simulink model "LCK_0112"  (R2018b)
settings: Solver=FixedStepDiscrete  StartTime=0.0  StopTime=inf  FixedStep=0.01  RelTol=1e-3
PostLoadFcn:
  | if any(exist('dsrtsu_mdlpostloadfcn', 'file') ~= 0), dsrtsu_mdlpostloadfcn('Execute', bdroot); end
values from neighbouring files (symbols this model uses):
  C_DEG2RAD = 0.0175    [LCK_Macro.sldd]
  C_KPH2MPS = 0.2778    [LCK_Macro.sldd]
  C_NEARZERO = 0.0001    [LCK_Macro.sldd]
  C_ONE = 1.0    [LCK_Macro.sldd]
  C_RAD2DEG = 57.2958    [LCK_Macro.sldd]
  C_ZERO = 0.0    [LCK_Macro.sldd]
  k_accel_pedal_pos_per_speed_x : value not decoded    [LCK_LogicPara.sldd]
  k_accel_pedal_pos_per_speed_z : value not decoded    [LCK_LogicPara.sldd]
  k_brake_suprress_hold = 1000.0    [LCK_LogicPara.sldd]
  k_driver_appl_torque_filt = 50.0    [LCK_LogicPara.sldd]
  k_driver_suppression_hold_time = 3000.0    [LCK_LogicPara.sldd]
  k_hands_on_wheel_hold_msec = 500.0    [LCK_LogicPara.sldd]
  k_hands_on_wheel_torque_hi = 0.2    [LCK_LogicPara.sldd]
  k_hands_on_wheel_torque_lo = 0.15    [LCK_LogicPara.sldd]
  k_handsoff_delay_cycles = 50.0    [LCK_LogicPara.sldd]
  k_handsoff_torq_Lo_CR = 0.3    [LCK_LogicPara.sldd]
  k_handson_delay_cycles = 5.0    [LCK_LogicPara.sldd]
  k_HighAccel_suppress_hold = 3000.0    [LCK_LogicPara.sldd]
  k_HLR_suprress_hold = 3000.0    [LCK_LogicPara.sldd]
  k_hs_StrAng_CR_threshold_z : value not decoded    [LCK_LogicPara.sldd]
  k_LC_Exit_Switch = 0.0    [LCK_LogicPara.sldd]
  k_LCG_Configured = 1.0    [LCK_LogicPara.sldd]
  k_LCK_A0_Rdy2Act_UseConst = 0.0    [LCK_LogicPara.sldd]
  k_LCK_A0Fac_ActSta : value not decoded    [LCK_CtrlPara.sldd]
  k_LCK_A0Fac_DrvStm : value not decoded    [LCK_CtrlPara.sldd]
  k_LCK_A0Shift_LftCurv : value not decoded    [LCK_CtrlPara.sldd]
  k_LCK_A0Shift_RgtCurv : value not decoded    [LCK_CtrlPara.sldd]
  k_LCK_A0Shift_StraLan = 0.0    [LCK_CtrlPara.sldd]
  k_LCK_A0ShiftFac_Dy_LftCurv : value not decoded    [LCK_CtrlPara.sldd]
  k_LCK_A0ShiftFac_Dy_RgtCurv : value not decoded    [LCK_CtrlPara.sldd]
  k_LCK_A0ShiftFac_Vspd : value not decoded    [LCK_CtrlPara.sldd]
  k_LCK_accel_inhibit_thold = 35.0    [LCK_LogicPara.sldd]
  k_LCK_Active2Ready_Mask = 255.0    [LCK_LogicPara.sldd]
  k_LCK_CvatRateBks : value not decoded    [LCK_CtrlPara.sldd]
  k_LCK_CvatrBks : value not decoded    [LCK_CtrlPara.sldd]
  k_LCK_DFac_Dy : value not decoded    [LCK_CtrlPara.sldd]
  k_LCK_DFac_Dy_Curv : value not decoded    [LCK_CtrlPara.sldd]
  k_LCK_DFac_HaCurCen : value not decoded    [LCK_CtrlPara.sldd]
  k_LCK_DFac_HaCurSid : value not decoded    [LCK_CtrlPara.sldd]
  k_LCK_DFac_HadCurCen : value not decoded    [LCK_CtrlPara.sldd]
  k_LCK_DFac_HadCurSid : value not decoded    [LCK_CtrlPara.sldd]
  k_LCK_DFac_HadStrCen : value not decoded    [LCK_CtrlPara.sldd]
  k_LCK_DFac_HadStrSid : value not decoded    [LCK_CtrlPara.sldd]
  k_LCK_DFac_HaStrCen : value not decoded    [LCK_CtrlPara.sldd]
  k_LCK_DFac_HaStrSid : value not decoded    [LCK_CtrlPara.sldd]
  k_LCK_DFac_Rad : value not decoded    [LCK_CtrlPara.sldd]
  k_LCK_DFac_SA_CurCen : value not decoded    [LCK_CtrlPara.sldd]
  k_LCK_DFac_SA_CurSid : value not decoded    [LCK_CtrlPara.sldd]
  k_LCK_DFac_SA_StrCen : value not decoded    [LCK_CtrlPara.sldd]
  k_LCK_DFac_SA_StrSid : value not decoded    [LCK_CtrlPara.sldd]
  k_LCK_DFac_SS_CurCen : value not decoded    [LCK_CtrlPara.sldd]
  k_LCK_DFac_SS_CurSid : value not decoded    [LCK_CtrlPara.sldd]
  k_LCK_DFac_SS_StrCen : value not decoded    [LCK_CtrlPara.sldd]
  k_LCK_DFac_SS_StrSid : value not decoded    [LCK_CtrlPara.sldd]
  k_LCK_DFac_Vspd : value not decoded    [LCK_CtrlPara.sldd]
  k_LCK_DlyTm_DrvStim = 0.2    [LCK_CtrlPara.sldd]
  k_LCK_DTermMax = 2.0    [LCK_CtrlPara.sldd]
  k_LCK_DyBks_Curv : value not decoded    [LCK_CtrlPara.sldd]
  k_LCK_Enable_POOnly = 1.0    [LCK_LogicPara.sldd]
  k_LCK_Entry_DistBuffer = 0.1    [LCK_LogicPara.sldd]
  k_LCK_Fac_Vspd2RngThr_FalRec = 0.23    [LCK_CtrlPara.sldd]
  k_LCK_Ffw_CvatSwh = 0.0    [LCK_CtrlPara.sldd]
  k_LCK_Ffw_DyBks : value not decoded    [LCK_CtrlPara.sldd]
  k_LCK_Ffw_TimCon_CmdFlt = 0.0    [LCK_CtrlPara.sldd]
  k_LCK_FfwDeltaFac_Rad_Lft : value not decoded    [LCK_CtrlPara.sldd]
  k_LCK_FfwDeltaFac_Rad_Rgt : value not decoded    [LCK_CtrlPara.sldd]
  k_LCK_FfwDeltaFac_Vspd : value not decoded    [LCK_CtrlPara.sldd]
  k_LCK_FfwFac_CvatRate_Lft : value not decoded    [LCK_CtrlPara.sldd]
  k_LCK_FfwFac_CvatRate_Rgt : value not decoded    [LCK_CtrlPara.sldd]
  k_LCK_FfwFac_Dy : value not decoded    [LCK_CtrlPara.sldd]
  k_LCK_FfwFac_Rad_Lft : value not decoded    [LCK_CtrlPara.sldd]
  k_LCK_FfwFac_Rad_Rgt : value not decoded    [LCK_CtrlPara.sldd]
  k_LCK_FfwFac_Vspd : value not decoded    [LCK_CtrlPara.sldd]
  k_LCK_FfwTorq_Cvat : value not decoded    [LCK_CtrlPara.sldd]
  k_LCK_HAFac_ActSta : value not decoded    [LCK_CtrlPara.sldd]
  k_LCK_HAFac_DrvStm : value not decoded    [LCK_CtrlPara.sldd]
  k_LCK_HaloTime = 2000.0    [LCK_LogicPara.sldd]
  k_LCK_HaloTime_Switch = 0.0    [LCK_LogicPara.sldd]
  k_LCK_HARFac_ActSta : value not decoded    [LCK_CtrlPara.sldd]
  k_LCK_HARFac_DrvStm : value not decoded    [LCK_CtrlPara.sldd]
  k_LCK_Hed_DyBks : value not decoded    [LCK_CtrlPara.sldd]
  k_LCK_HedAngDiffX : value not decoded    [LCK_CtrlPara.sldd]
  k_LCK_HedAngRateDiffX : value not decoded    [LCK_CtrlPara.sldd]
  k_LCK_HndsOnWhel_DlyTm_Idl2Rdy = 0.0    [LCK_LogicPara.sldd]
  k_LCK_host_veh_width = 1.86    [LCK_LogicPara.sldd]
  k_LCK_Idle2Ready_Mask = 239.0    [LCK_LogicPara.sldd]
  k_LCK_Junc_SusTime = 1.0    [LCK_LogicPara.sldd]
  k_LCK_KpKdDecSlopeLmt = 10.0    [LCK_CtrlPara.sldd]
  k_LCK_KpKdIncSlopeLmt = 5.0    [LCK_CtrlPara.sldd]
  k_LCK_Lat_Ctrl_DFac_Lft = 1.0    [LCK_CtrlPara.sldd]
  k_LCK_Lat_Ctrl_DFac_Rgt = 1.05    [LCK_CtrlPara.sldd]
  k_LCK_Lat_Ctrl_Kd = 0.8    [LCK_CtrlPara.sldd]
  k_LCK_Lat_Ctrl_Ki = 0.5    [LCK_CtrlPara.sldd]
  k_LCK_Lat_Ctrl_Kp = 0.7    [LCK_CtrlPara.sldd]
  k_LCK_Lat_Ctrl_Kp_NearGain = 0.7    [LCK_CtrlPara.sldd]
  k_LCK_Lat_Ctrl_PFac_Lft = 1.0    [LCK_CtrlPara.sldd]
  k_LCK_Lat_Ctrl_PFac_Rgt = 1.05    [LCK_CtrlPara.sldd]
  k_LCK_Lat_Ctrl_TimCon_CmdFlt = 5.0    [LCK_CtrlPara.sldd]
  k_LCK_Lat_DFac_Rad : value not decoded    [LCK_CtrlPara.sldd]
  k_LCK_Lat_DFac_SS_Cur : value not decoded    [LCK_CtrlPara.sldd]
  k_LCK_Lat_DFac_SS_Str : value not decoded    [LCK_CtrlPara.sldd]
  k_LCK_Lat_DFac_Vspd : value not decoded    [LCK_CtrlPara.sldd]
  k_LCK_Lat_DyBks : value not decoded    [LCK_CtrlPara.sldd]
  k_LCK_Lat_IFac_Rad : value not decoded    [LCK_CtrlPara.sldd]
  k_LCK_Lat_IFac_Vspd : value not decoded    [LCK_CtrlPara.sldd]
  k_LCK_Lat_ILmtFac_Dy_CurvLan : value not decoded    [LCK_CtrlPara.sldd]
  k_LCK_Lat_ILmtFac_Dy_StraLan : value not decoded    [LCK_CtrlPara.sldd]
  k_LCK_Lat_ILmtFac_Rad : value not decoded    [LCK_CtrlPara.sldd]
  k_LCK_Lat_ILmtFac_Rad_NearGain = 1.0    [LCK_CtrlPara.sldd]
  k_LCK_Lat_ILmtFac_Vspd_CurvLan : value not decoded    [LCK_CtrlPara.sldd]
  k_LCK_Lat_ILmtFac_Vspd_StraLan : value not decoded    [LCK_CtrlPara.sldd]
  k_LCK_Lat_ITermLmt_Dy = 1.0    [LCK_CtrlPara.sldd]
  k_LCK_Lat_KpKdDecSlopeLmt = 10.0    [LCK_CtrlPara.sldd]
  k_LCK_Lat_KpKdIncSlopeLmt = 10.0    [LCK_CtrlPara.sldd]
  k_LCK_Lat_PFac_Dy_InnLftCur : value not decoded    [LCK_CtrlPara.sldd]
  k_LCK_Lat_PFac_Dy_InnRgtCur : value not decoded    [LCK_CtrlPara.sldd]
  k_LCK_Lat_PFac_Dy_OutLftCur : value not decoded    [LCK_CtrlPara.sldd]
  k_LCK_Lat_PFac_Dy_OutRgtCur : value not decoded    [LCK_CtrlPara.sldd]
  k_LCK_Lat_PFac_Dy_Str : value not decoded    [LCK_CtrlPara.sldd]
  k_LCK_Lat_PFac_Rad : value not decoded    [LCK_CtrlPara.sldd]
  ... (+153 more)
undefined symbols (not defined in the file or in its folder): k_LCK_CurvBks, K_LCK_SPA0A1A2_LMRngCmp_y
libraries: LateralControl_fcns_lib x58, simulink x24
(part 5 of 45)

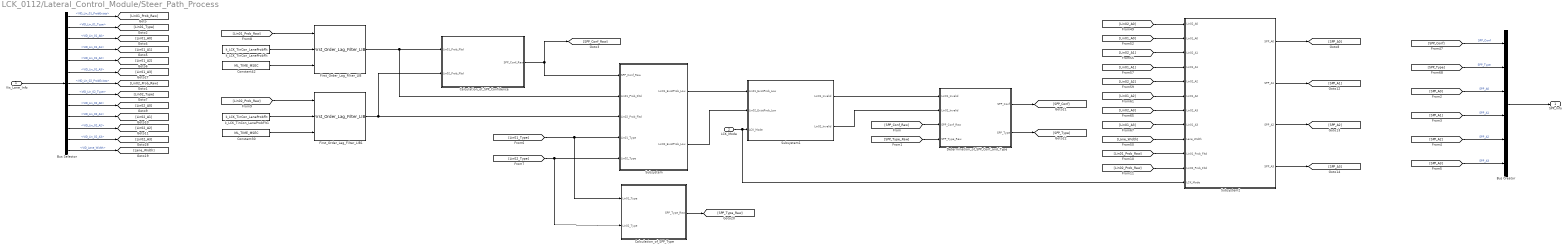
== system LCK_0112/Lateral_Control_Module/Steer_Path_Process ==
  Vis_Lane_Info : Inport  Description=_GWMH9P3.Latctrl.000_23_
  LCK_Mode : Inport  Description=_GWMH9P3.Latctrl.000_23_  Port=2
  Bus Creator : BusCreator  Inputs=6  OutDataTypeStr=Bus: LatCtrl_LCK_SPPInfo_t
      settings: InheritFromInputs=off
  Bus Selector : BusSelector  OutputSignals=VID_Lin_01_ProbExists,VID_Lin_01_Type,VID_Lin_01_A0,VID_Lin_01_A1,VID_Lin_01_A2,VID_Lin_01_A3,VID_Lin_02_ProbExists,VID_Lin_02_Type,VID_Lin_02_A0,VID_Lin_02_A1,VID_Lin_02_A2,VID_Lin_02_A3,VID_Lane_Width
  Calculation_of_SPP_Confidence : Subsystem
  Calculation_of_SPP_Type : Subsystem
  Constant30 : Constant  Tag={'output',{'name','$P','class','EXTERN_MACRO','type','ESR_Typedefs/unsigned8_T'},'date',737462.69417376153}  Description=_GWMH9P4.LCK.000_202_  Value=ML_TIME_MSEC
  Constant42 : Constant  Tag={'output',{'name','$P','class','EXTERN_MACRO','type','ESR_Typedefs/unsigned8_T'},'date',737462.69417376153}  Description=_GWMH9P4.LCK.000_202_  Value=ML_TIME_MSEC
  Determination_of_SPP_Conf_and_Type : Subsystem
  First_Order_Lag_Filter_LIB : LateralControl_fcns_lib/First_Order_Lag_Filter_LIB  SystemSampleTime=-1
  First_Order_Lag_Filter_LIB1 : LateralControl_fcns_lib/First_Order_Lag_Filter_LIB  SystemSampleTime=-1
  Subsystem : Subsystem
  Subsystem1 : Subsystem
  Subsystem2 : Subsystem
  k_LCK_TinCon_LaneProbFlt : Constant  Tag={'output',{'name','$P','class','EXTERN_MACRO','type','ESR_Typedefs/unsigned8_T'},'date',737462.69417376153}  Description=_GWMH9P4.LCK.000_202_  Value=k_LCK_TinCon_LaneProbFlt
  k_LCK_TinCon_LaneProbFlt1 : Constant  Tag={'output',{'name','$P','class','EXTERN_MACRO','type','ESR_Typedefs/unsigned8_T'},'date',737462.69417376153}  Description=_GWMH9P4.LCK.000_202_  Value=k_LCK_TinCon_LaneProbFlt
  SPP_Info : Outport
  wires:
  Vis_Lane_Info/1 -> Bus Selector/1
  Bus Selector/1 -> [Lin01_Prob_Raw]  "<VID_Lin_01_ProbExists>"
  Bus Selector/2 -> [Lin01_Type]  "<VID_Lin_01_Type>"
  Bus Selector/3 -> [Lin01_A0]  "<VID_Lin_01_A0>"
  Bus Selector/4 -> [Lin01_A1]  "<VID_Lin_01_A1>"
  Bus Selector/5 -> [Lin01_A2]  "<VID_Lin_01_A2>"
  Bus Selector/7 -> [Lin02_Prob_Raw]  "<VID_Lin_02_ProbExists>"
  Bus Selector/8 -> [Lin02_Type]  "<VID_Lin_02_Type>"
  Bus Selector/9 -> [Lin02_A0]  "<VID_Lin_02_A0>"
  Bus Selector/10 -> [Lin02_A1]  "<VID_Lin_02_A1>"
  Bus Selector/11 -> [Lin02_A2]  "<VID_Lin_02_A2>"
  k_LCK_TinCon_LaneProbFlt/1 -> First_Order_Lag_Filter_LIB/2
  Constant42/1 -> First_Order_Lag_Filter_LIB/3
  [Lin01_Prob_Raw] -> First_Order_Lag_Filter_LIB/1
  [Lin02_Prob_Raw] -> First_Order_Lag_Filter_LIB1/1
  Constant30/1 -> First_Order_Lag_Filter_LIB1/3
  k_LCK_TinCon_LaneProbFlt1/1 -> First_Order_Lag_Filter_LIB1/2
  Bus Selector/13 -> [Lane_Width]  "<VID_Lane_Width>"
  [SPP_Conf] -> Bus Creator/1  "SPP_Conf"
  [SPP_Type] -> Bus Creator/2  "SPP_Type"
  Bus Creator/1 -> SPP_Info/1
  Bus Selector/6 -> [Lin01_A3]  "<VID_Lin_01_A3>"
  Bus Selector/12 -> [Lin02_A3]  "<VID_Lin_02_A3>"
  First_Order_Lag_Filter_LIB/1 -> Calculation_of_SPP_Confidence/1(Lin01_Prob_Fltd), Subsystem/2(Lin01_Prob_Fltd)
  First_Order_Lag_Filter_LIB1/1 -> Subsystem/3(Lin02_Prob_Fltd), Calculation_of_SPP_Confidence/2(Lin02_Prob_Fltd)
  Calculation_of_SPP_Confidence/1(SPP_Conf_Raw) -> [SPP_Conf_Raw], Subsystem/1(SPP_Conf_Raw)
  [Lin01_Type] -> Calculation_of_SPP_Type/1(Lin01_Type), Subsystem/4(Lin01_Type)
  [Lin02_Type] -> Calculation_of_SPP_Type/2(Lin02_Type), Subsystem/5(Lin02_Type)
  Calculation_of_SPP_Type/1(SPP_Type_Raw) -> [SPP_Type_Raw]
  LCK_Mode/1 -> Subsystem2/12(LCK_Mode), Subsystem1/3(LCK_Mode)
  Subsystem1/1(Lin01_Invalid) -> Determination_of_SPP_Conf_and_Type/1(Lin01_Invalid)
  Subsystem1/2(Lin02_Invalid) -> Determination_of_SPP_Conf_and_Type/2(Lin02_Invalid)
  Subsystem/1(Lin01_ExistProb_Low) -> Subsystem1/1(Lin01_ExistProb_Low)
  Subsystem/2(Lin02_ExistProb_Low) -> Subsystem1/2(Lin02_ExistProb_Low)
  Determination_of_SPP_Conf_and_Type/1(SPP_Conf) -> [SPP_Conf]
  Determination_of_SPP_Conf_and_Type/2(SPP_Type) -> [SPP_Type]
  [Lin02_A0] -> Subsystem2/1(Lin02_A0)
  [Lin01_A0] -> Subsystem2/2(Lin01_A0)
  [Lin02_A1] -> Subsystem2/3(Lin02_A1)
  [Lin01_A1] -> Subsystem2/4(Lin01_A1)
  [Lin02_A2] -> Subsystem2/5(Lin02_A2)
  [Lin01_A2] -> Subsystem2/6(Lin01_A2)
  [Lane_Width] -> Subsystem2/9(Lane_Width)
  [Lin02_A3] -> Subsystem2/7(Lin02_A3)
  [Lin01_A3] -> Subsystem2/8(Lin01_A3)
  [SPP_Conf_Raw] -> Determination_of_SPP_Conf_and_Type/3(SPP_Conf_Raw)
  [SPP_Type_Raw] -> Determination_of_SPP_Conf_and_Type/4(SPP_Type_Raw)
  [SPP_A0] -> Bus Creator/3  "SPP_A0"
  [SPP_A1] -> Bus Creator/4  "SPP_A1"
  [SPP_A2] -> Bus Creator/5  "SPP_A2"
  [SPP_A3] -> Bus Creator/6  "SPP_A3"
  Subsystem2/1(SPP_A0) -> [SPP_A0]
  Subsystem2/2(SPP_A1) -> [SPP_A1]
  Subsystem2/3(SPP_A2) -> [SPP_A2]
  Subsystem2/4(SPP_A3) -> [SPP_A3]
  [Lin01_Prob_Raw] -> Subsystem2/10(Lin01_Prob_Fltd)
  [Lin02_Prob_Raw] -> Subsystem2/11(Lin02_Prob_Fltd)

== system LCK_0112/RTI Data/RTI Data Store ==
  RTI Data Store : Subsystem  mask(RTI_DATA_STORE){}
      mask help:
      | RTI Data Store Block. This block is used by RTI to store internal model dependent data. Deleting this block will result in data loss.
      |
      | NEVER DELETE, COPY, OR MODIFY THIS BLOCK!
      mask Help:
      | RTI Data Store Block. This block is used by RTI to store internal model dependent data. Deleting this block will result in data loss.
      | 
      | NEVER DELETE, COPY, OR MODIFY THIS BLOCK!
      mask Display: text(0.5, 0.5, ' ', 'HorizontalAlignment', 'center');

== system LCK_0112/Lateral_Control_Module/Adas_Lateral_Control_LCK_Core/Lateral Control State Detection ==
  LCK_Mode : Inport  Description=_GWMAB30P4.LCK.000_293_
  Constant1 : Constant  Description=_GWMAB30P3.LCK.000_155_  Value=2  OutDataTypeStr=uint8
  Constant2 : Constant  Description=_GWMAB30P3.LCK.000_155_  Value=0  OutDataTypeStr=uint8
  Constant3 : Constant  Description=_GWMAB30P3.LCK.000_155_  Value=3  OutDataTypeStr=uint8
  Constant4 : Constant  Description=_GWMAB30P3.LCK.000_155_  OutDataTypeStr=uint8
  LCK_MODE_ACTIVE : Constant  Tag={'output',{'name','$P','max',23,'min',0,'class','EXTERN_MACRO','type','UInt8','scaling','VOID_SCALING'},'date',737296.63830359955}  Description=_GWMAB30P2.LCK.000_1337_  Value=LCK_MODE_ACTIVE
  LCK_MODE_LEFT_LANE_CHANGE : Constant  Tag={'output',{'name','$P','max',23,'min',0,'class','EXTERN_MACRO','type','UInt8','scaling','VOID_SCALING'},'date',737296.63830359955}  Description=_GWMAB30P2.LCK.000_1337_  Value=LCK_MODE_LEFT_LANE_CHANGE
  LCK_MODE_RIGHT_LANE_CHANGE : Constant  Tag={'output',{'name','$P','max',23,'min',0,'class','EXTERN_MACRO','type','UInt8','scaling','VOID_SCALING'},'date',737296.63830359955}  Description=_GWMAB30P2.LCK.000_1337_  Value=LCK_MODE_RIGHT_LANE_CHANGE
  Relational Operator1 : RelationalOperator  Tag={'date',737184.60401761578}  Description=_GWMAB30P2.LCK.000_1388_  Operator===  RndMeth=Nearest
  Relational Operator16 : RelationalOperator  Tag={'date',737184.60401761578}  Description=_GWMAB30P2.LCK.000_1388_  RndMeth=Nearest
  Relational Operator2 : RelationalOperator  Tag={'date',737184.60401761578}  Description=_GWMAB30P2.LCK.000_1388_  Operator===  RndMeth=Nearest
  Switch : Switch  Description=_GWMAB30P2.LCK.000_1368_  Threshold=0.5
  Switch1 : Switch  Description=_GWMAB30P2.LCK.000_1368_  Threshold=0.5
  Switch2 : Switch  Description=_GWMAB30P2.LCK.000_1368_  Threshold=0.5
  Lat_Ctrl_State : Outport
  wires:
  LCK_Mode/1 -> Relational Operator16/1, Relational Operator1/1, Relational Operator2/1
  LCK_MODE_ACTIVE/1 -> Relational Operator16/2
  Relational Operator16/1 -> Switch/2
  Constant2/1 -> Switch/3
  Switch/1 -> Lat_Ctrl_State/1
  LCK_MODE_LEFT_LANE_CHANGE/1 -> Relational Operator1/2
  Relational Operator1/1 -> Switch1/2
  Constant1/1 -> Switch1/1
  LCK_MODE_RIGHT_LANE_CHANGE/1 -> Relational Operator2/2
  Relational Operator2/1 -> Switch2/2
  Constant3/1 -> Switch2/1
  Switch2/1 -> Switch1/3
  Switch1/1 -> Switch/1
  Constant4/1 -> Switch2/3
